simulink model "sympathetic_trip"  (R2019b)
settings: Solver=FixedStepAuto  StartTime=0.0  StopTime=1  FixedStep=0.0001  RelTol=1e-3
libraries: powerlib x16, powerlib_meascontrol x10, simulink x3, artemis x3
settings Model: Creator=nikgal-local  LastModifiedBy=nikgal-local
settings DataIOCC: ReturnWorkspaceOutputs=off
settings DebuggingCC: UnconnectedInputMsg=none  UnconnectedOutputMsg=none  UnconnectedLineMsg=none
settings RTWCC: GenCodeOnly=on

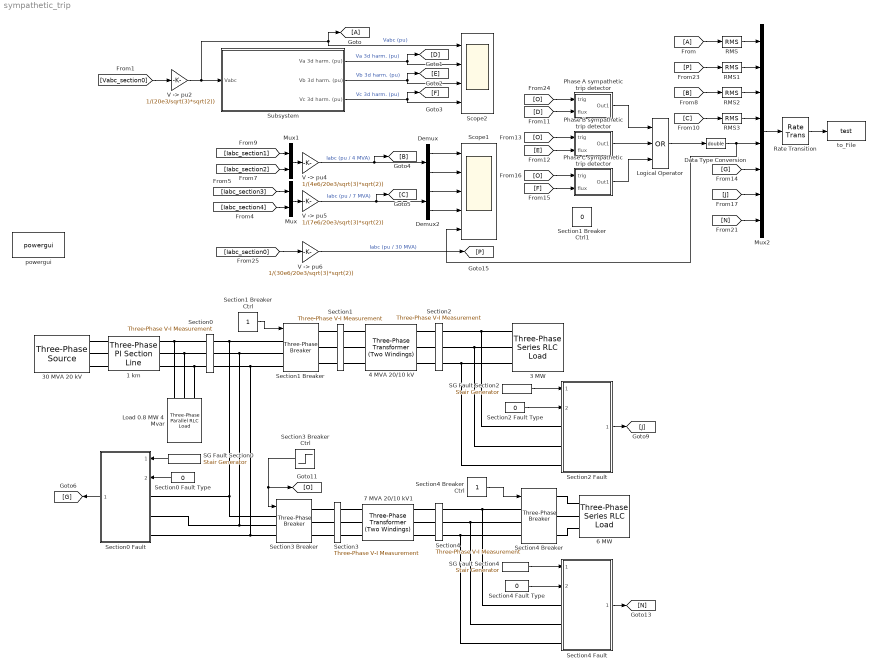
== system sympathetic_trip ==
  1 km : powerlib/Elements/Three-Phase PI Section Line  LConnTagsString=a|b|c  RConnTagsString=A|B|C  Frequency=50  Resistances=[ 0.01273 0.3864]  Inductances="[ 0.9337e-3  4.1264e-3]"  Capacitances=[12.74e-9 7.751e-9]  Length=1
      settings: SourceProductName=Simscape Electrical
  3 MW : powerlib/Elements/Three-Phase Series RLC Load  LConnTagsString=A|B|C  Configuration=Y (grounded)  NominalVoltage=10e3  Vabc=[1e3 1e3 1e3]  Vabcp=[1e3 1e3 1e3]  NominalFrequency=50  UnbalancedPower=off  ActivePower=3e6  InductivePower=0  CapacitivePower=0  Pabc=[10e3 9e3 11e3]  QLabc=[100 90 110]  QCabc=[100 90 110]  Pabcp=[10e3 9e3 11e3]  QLabcp=[100 90 110]  QCabcp=[100 90 110]  Measurements=None  LoadType=constant Z
      settings: SourceProductName=Simscape Electrical
  30 MVA 20 kV : powerlib/Electrical Sources/Three-Phase Source  InternalConnection=Yg  VoltagePhases=off  Voltage=20e3  PhaseAngle=15  Voltage_phases=[25e3 25e3 25e3]/sqrt(3)  PhaseAngles_phases=[0 -120 +120]  Frequency=50  NonIdealSource=on  SpecifyImpedance=off  Resistance=1.33  Inductance=35.3e-3  ShortCircuitLevel=30e6  BaseVoltage=20e3  XRratio=10  BusType=swing  Pref=10e3  Qref=0  Prefabc=[10e3, 10e3, 10e3]  Qrefabc=[0, 0, 0]  Qmin=-inf  Qmax=inf
      settings: SourceProductName=Simscape Electrical
  4 MVA 20/10 kV : powerlib/Elements/Three-Phase Transformer (Two Windings)  Winding1Connection=Yg  Winding2Connection=Yg  CoreType=Three single-phase transformers  SetSaturation=on  Hysteresis=off  DataFile='hysteresis'  SetInitialFlux=off  Measurements=None  UNITS=pu  NominalPower=[ 4e6 , 50 ]  Winding1=[ 20e3 , 0.05 , 0.08 ]  Winding2=[ 10e3 , 0.05 , 0.08 ]  Rm=500  Lm=500  L0=0.5  Saturation=[ 0,0 ; 0.0012,1.2 ; 1.0,1.45 ]  InitialFluxes=[-1.04733441543709 0.447873926928996 0.599252337980466]  BreakLoop=off  DiscreteSolver=Trapezoidal iterative  DataType=off  TransfoNumber=1
      settings: SourceProductName=Simscape Electrical
  6 MW : powerlib/Elements/Three-Phase Series RLC Load  LConnTagsString=A|B|C  Configuration=Y (grounded)  NominalVoltage=10e3  Vabc=[1e3 1e3 1e3]  Vabcp=[1e3 1e3 1e3]  NominalFrequency=50  UnbalancedPower=off  ActivePower=6e6  InductivePower=0  CapacitivePower=0  Pabc=[10e3 9e3 11e3]  QLabc=[100 90 110]  QCabc=[100 90 110]  Pabcp=[10e3 9e3 11e3]  QLabcp=[100 90 110]  QCabcp=[100 90 110]  Measurements=None  LoadType=constant Z
      settings: SourceProductName=Simscape Electrical
  7 MVA 20/10 kV1 : powerlib/Elements/Three-Phase Transformer (Two Windings)  Winding1Connection=Yg  Winding2Connection=Yg  CoreType=Three single-phase transformers  SetSaturation=on  Hysteresis=off  DataFile='hysteresis'  SetInitialFlux=on  Measurements=None  UNITS=pu  NominalPower=[ 7e6 , 50 ]  Winding1=[ 20e3 , 0.05 , 0.08 ]  Winding2=[ 10e3 , 0.05 , 0.08 ]  Rm=500  Lm=500  L0=0.5  Saturation=[ 0,0 ; 0.0012,1.2 ; 1.0,1.45 ]  InitialFluxes=[0.8 -0.4 0.4]  BreakLoop=off  DiscreteSolver=Trapezoidal iterative  DataType=off  TransfoNumber=1
      settings: SourceProductName=Simscape Electrical
  Data Type Conversion : DataTypeConversion  OutMin=[0]  OutMax=[1]  OutDataTypeStr=double
  Demux : Demux  Outputs=2
  Demux2 : Demux  Outputs=2
  Load 0.8 MW 4 Mvar : powerlib/Elements/Three-Phase Parallel RLC Load  LConnTagsString=A|B|C  Configuration=Y (grounded)  NominalVoltage=20e3  Vabc=[1e3 1e3 1e3]  Vabcp=[1e3 1e3 1e3]  NominalFrequency=50  UnbalancedPower=off  ActivePower=0.8e6  InductivePower=0  CapacitivePower=4e6  Pabc=[10e3 9e3 11e3]  QLabc=[100 90 110]  QCabc=[100 90 110]  Pabcp=[10e3 9e3 11e3]  QLabcp=[100 90 110]  QCabcp=[100 90 110]  Measurements=None  LoadType=constant Z
      settings: SourceProductName=Simscape Electrical
  Logical Operator : Logic  Operator=OR  Inputs=3  AllPortsSameDT=off  OutDataTypeStr=boolean
  Mux : Mux  Inputs=2
  Mux1 : Mux  Inputs=2
  Mux2 : Mux  Inputs=8
  Phase A sympathetic trip detector : Subsystem
  Phase B sympathetic trip detector : Subsystem
  Phase C sympathetic trip detector : Subsystem
  RMS{,1..3} (4 alike) : powerlib_meascontrol/Measurements/RMS  TrueRMS=on  Freq=50  RMSInit=1  Ts=0
      settings: SourceProductName=Simscape Electrical
  Rate Transition : RateTransition  OutPortSampleTime=0.0005
  SG Fault Section0 : powerlib_meascontrol/Pulse & Signal Generators/Stair Generator  t=[0, 0.5, 0.7]  e=[0, 1, 0]  Ts=0
      settings: SourceProductName=Simscape Electrical
  SG Fault Section2 : powerlib_meascontrol/Pulse & Signal Generators/Stair Generator  t=[0, 0.5, 0.7]  e=[0, 1, 0]  Ts=0
      settings: SourceProductName=Simscape Electrical
  SG Fault Section4 : powerlib_meascontrol/Pulse & Signal Generators/Stair Generator  t=[0, 0.5, 0.7]  e=[0, 1, 0]  Ts=0
      settings: SourceProductName=Simscape Electrical
  Scope1 : Scope  NumInputPorts=5
  Scope2 : Scope  NumInputPorts=4
  Section0 : powerlib/Measurements/Three-Phase V-I Measurement  VoltageMeasurement=phase-to-ground  SetLabelV=on  LabelV=Vabc_section0  Vpu=off  VpuLL=off  CurrentMeasurement=yes  SetLabelI=on  LabelI=Iabc_section0  Ipu=off  Pbase=100e6  Vbase=500e3  OutputType=Complex  PhasorSimulation=off  PSBequivalent=0
      settings: SourceProductName=Simscape Electrical
  Section0 Fault : Subsystem
  Section0 Fault Type : Constant  Value=0
  Section1 : powerlib/Measurements/Three-Phase V-I Measurement  VoltageMeasurement=phase-to-ground  SetLabelV=on  LabelV=Vabc_section1  Vpu=off  VpuLL=off  CurrentMeasurement=yes  SetLabelI=on  LabelI=Iabc_section1  Ipu=off  Pbase=100e6  Vbase=500e3  OutputType=Complex  PhasorSimulation=off  PSBequivalent=0
      settings: SourceProductName=Simscape Electrical
  Section1 Breaker : powerlib/Elements/Three-Phase Breaker  InitialState=closed  SwitchA=on  SwitchB=on  SwitchC=on  SwitchTimes=[0]  External=on  BreakerResistance=0.01  SnubberResistance=1e6  SnubberCapacitance=150e-6  Measurements=None
      settings: SourceProductName=Simscape Electrical
  Section1 Breaker Ctrl : Constant
  Section1 Breaker Ctrl1 : Constant  Value=0
  Section2 : powerlib/Measurements/Three-Phase V-I Measurement  VoltageMeasurement=no  SetLabelV=off  LabelV=Vabc  Vpu=off  VpuLL=off  CurrentMeasurement=yes  SetLabelI=on  LabelI=Iabc_section2  Ipu=off  Pbase=100e6  Vbase=500e3  OutputType=Complex  PhasorSimulation=off  PSBequivalent=0
      settings: SourceProductName=Simscape Electrical
  Section2 Fault : Subsystem
  Section2 Fault Type : Constant  Value=0
  Section3 : powerlib/Measurements/Three-Phase V-I Measurement  VoltageMeasurement=no  SetLabelV=off  LabelV=Vabc  Vpu=off  VpuLL=off  CurrentMeasurement=yes  SetLabelI=on  LabelI=Iabc_section3  Ipu=off  Pbase=100e6  Vbase=500e3  OutputType=Complex  PhasorSimulation=off  PSBequivalent=0
      settings: SourceProductName=Simscape Electrical
  Section3 Breaker : powerlib/Elements/Three-Phase Breaker  InitialState=open  SwitchA=on  SwitchB=on  SwitchC=on  SwitchTimes=[12/50]  External=on  BreakerResistance=0.01  SnubberResistance=1e6  SnubberCapacitance=150e-6  Measurements=None
      settings: SourceProductName=Simscape Electrical
  Section3 Breaker Ctrl : Step  Time=0.5  SampleTime=0
  Section4 : powerlib/Measurements/Three-Phase V-I Measurement  VoltageMeasurement=no  SetLabelV=off  LabelV=Vabc  Vpu=off  VpuLL=off  CurrentMeasurement=yes  SetLabelI=on  LabelI=Iabc_section4  Ipu=off  Pbase=100e6  Vbase=500e3  OutputType=Complex  PhasorSimulation=off  PSBequivalent=0
      settings: SourceProductName=Simscape Electrical
  Section4 Breaker : powerlib/Elements/Three-Phase Breaker  InitialState=closed  SwitchA=on  SwitchB=on  SwitchC=on  SwitchTimes=[12/50]  External=on  BreakerResistance=0.01  SnubberResistance=1e6  SnubberCapacitance=150e-6  Measurements=None
      settings: SourceProductName=Simscape Electrical
  Section4 Breaker Ctrl : Constant
  Section4 Fault : Subsystem
  Section4 Fault Type : Constant  Value=0
  Subsystem : Subsystem
  "V -> pu2" : Gain  Gain=1/(20e3/sqrt(3)*sqrt(2))  SaturateOnIntegerOverflow=on  OutDataTypeStr=Inherit: Same as input  ParamDataTypeStr=Inherit: Same as input
  "V -> pu4" : Gain  Gain=1/(4e6/20e3/sqrt(3)*sqrt(2))  SaturateOnIntegerOverflow=on  OutDataTypeStr=Inherit: Same as input  ParamDataTypeStr=Inherit: Same as input
  "V -> pu5" : Gain  Gain=1/(7e6/20e3/sqrt(3)*sqrt(2))  SaturateOnIntegerOverflow=on  OutDataTypeStr=Inherit: Same as input  ParamDataTypeStr=Inherit: Same as input
  "V -> pu6" : Gain  Gain=1/(30e6/20e3/sqrt(3)*sqrt(2))  SaturateOnIntegerOverflow=on  OutDataTypeStr=Inherit: Same as input  ParamDataTypeStr=Inherit: Same as input
  powergui : powerlib/powergui  Priority=1  SimulationMode=Discrete  SampleTime=0.0001  frequency=60  Iterations=50  frequencyindice=0  Pbase=100e6  ErrMax=1e-4  UnitsV=kV  UnitsW=MW  buscounter=0  FunctionMessages=off  echomessages=off  EnableUseOfTLC=off  CurrentSourceSwitches=off  DisableSnubberDevices=off  DisableRonSwitches=off  DisableVfSwitches=off  DisplayEquations=off  AutomaticDiscreteSolvers=off  SolverType=Tustin/Backward Euler (TBE)  Interpol=off  ExternalGateDelay=off  methode=off  Ts=100  x0status=blocks  SPID=on  SwTol=0  HookPort=off  NonlinearTolerance=1e-4  nMaxIteration=100  ContinueOnMaxIteration=off  RestoreLinks=warning  ResistiveCurrentMeasurement=off  Frange=[0:2:500]  Ylog=off  Xlog=on  ShowGrid=off  save=off  variable=ZData  structure=my_test_scope1  ZoomFFT=off  StartTime=0.33  cycles=4  DisplayStyle=1  fundamental=50  FreqAxis=on  MaxFrequency=1000  frequencyindicesteady=1  RmsSteady=1  display=off
      settings: SourceProductName=Simscape Electrical
  to_File : ToFile  Filename=test
  wires:
  "V -> pu2"/1 -> [A], Scope2/1, Subsystem/1(Vabc)  "Vabc (pu)"
  [Vabc_section0] -> "V -> pu2"/1
  Subsystem/1(Va 3d harm. (pu)) -> [D], Scope2/2  "Va 3d harm. (pu)"
  Subsystem/2(Vb 3d harm. (pu)) -> [E], Scope2/3  "Vb 3d harm. (pu)"
  Subsystem/3(Vc 3d harm. (pu)) -> [F], Scope2/4  "Vc 3d harm. (pu)"
  [Iabc_section3] -> Mux/1
  [Iabc_section4] -> Mux/2
  Mux/1 -> "V -> pu5"/1
  Mux1/1 -> "V -> pu4"/1
  "V -> pu4"/1 -> [B], Demux/1  "Iabc (pu / 4 MVA)"
  [Iabc_section1] -> Mux1/1
  [Iabc_section2] -> Mux1/2
  "V -> pu5"/1 -> [C], Demux2/1  "Iabc (pu / 7 MVA)"
  Demux/1 -> Scope1/1
  Demux/2 -> Scope1/2
  Demux2/1 -> Scope1/3
  Demux2/2 -> Scope1/4
  [A] -> RMS/1
  Section3 Breaker Ctrl/1 -> [O], Section3 Breaker/1
  Section4 Breaker Ctrl/1 -> Section4 Breaker/1
  "V -> pu6"/1 -> [P]  "Iabc (pu / 30 MVA)"
  [Iabc_section0] -> "V -> pu6"/1
  [P] -> RMS1/1
  [B] -> RMS2/1
  [C] -> RMS3/1
  [O] -> Phase A sympathetic trip detector/1(trig)
  [D] -> Phase A sympathetic trip detector/2(flux)
  [O] -> Phase B sympathetic trip detector/1(trig)
  [E] -> Phase B sympathetic trip detector/2(flux)
  [F] -> Phase C sympathetic trip detector/2(flux)
  [O] -> Phase C sympathetic trip detector/1(trig)
  Mux2/1 -> Rate Transition/1
  Rate Transition/1 -> to_File/1
  RMS/1 -> Mux2/1
  RMS1/1 -> Mux2/2
  RMS2/1 -> Mux2/3
  RMS3/1 -> Mux2/4
  Section1 Breaker Ctrl/1 -> Section1 Breaker/1
  Phase A sympathetic trip detector/1(Out1) -> Logical Operator/1
  Phase B sympathetic trip detector/1(Out1) -> Logical Operator/2
  Phase C sympathetic trip detector/1(Out1) -> Logical Operator/3
  [G] -> Mux2/6
  [J] -> Mux2/7
  [N] -> Mux2/8
  Logical Operator/1 -> Data Type Conversion/1
  Data Type Conversion/1 -> Scope1/5, Mux2/5
  SG Fault Section2/1 -> Section2 Fault/1(activate fault)
  Section2 Fault/1(fault status) -> [J]
  Section2 Fault Type/1 -> Section2 Fault/2(fault type)
  SG Fault Section0/1 -> Section0 Fault/1(activate fault)
  Section0 Fault Type/1 -> Section0 Fault/2(fault type)
  Section0 Fault/1(fault status) -> [G]
  Section4 Fault/1(fault status) -> [N]
  Section4 Fault Type/1 -> Section4 Fault/2(fault type)
  SG Fault Section4/1 -> Section4 Fault/1(activate fault)
  connections:
  30 MVA 20 kV/RConn2 -- 1 km/LConn2
  30 MVA 20 kV/RConn1 -- 1 km/LConn1
  30 MVA 20 kV/RConn3 -- 1 km/LConn3
  Section1 Breaker/LConn1 -- Section3 Breaker/LConn1 -- Section0 Fault/LConn1 -- Section0/RConn1
  Section3 Breaker/LConn2 -- Section0 Fault/LConn2 -- Section1 Breaker/LConn2 -- Section0/RConn2
  Section1 Breaker/LConn3 -- Section0 Fault/LConn3 -- Section3 Breaker/LConn3 -- Section0/RConn3
  4 MVA 20/10 kV/RConn1 -- Section2/LConn1
  4 MVA 20/10 kV/RConn2 -- Section2/LConn2
  4 MVA 20/10 kV/RConn3 -- Section2/LConn3
  3 MW/LConn1 -- Section2 Fault/LConn1 -- Section2/RConn1
  3 MW/LConn2 -- Section2 Fault/LConn2 -- Section2/RConn2
  3 MW/LConn3 -- Section2 Fault/LConn3 -- Section2/RConn3
  Section3 Breaker/RConn1 -- Section3/LConn1
  Section3 Breaker/RConn2 -- Section3/LConn2
  Section3 Breaker/RConn3 -- Section3/LConn3
  7 MVA 20/10 kV1/LConn1 -- Section3/RConn1
  7 MVA 20/10 kV1/LConn2 -- Section3/RConn2
  7 MVA 20/10 kV1/LConn3 -- Section3/RConn3
  7 MVA 20/10 kV1/RConn1 -- Section4/LConn1
  7 MVA 20/10 kV1/RConn2 -- Section4/LConn2
  7 MVA 20/10 kV1/RConn3 -- Section4/LConn3
  Section4 Breaker/LConn3 -- Section4 Fault/LConn3 -- Section4/RConn3
  6 MW/LConn3 -- Section4 Breaker/RConn3
  6 MW/LConn2 -- Section4 Breaker/RConn2
  6 MW/LConn1 -- Section4 Breaker/RConn1
  Section4 Breaker/LConn2 -- Section4 Fault/LConn2 -- Section4/RConn2
  Section4 Breaker/LConn1 -- Section4 Fault/LConn1 -- Section4/RConn1
  Section1/RConn1 -- 4 MVA 20/10 kV/LConn1
  Section1/RConn2 -- 4 MVA 20/10 kV/LConn2
  Section1/RConn3 -- 4 MVA 20/10 kV/LConn3
  Section1 Breaker/RConn1 -- Section1/LConn1
  Section1 Breaker/RConn2 -- Section1/LConn2
  Section1 Breaker/RConn3 -- Section1/LConn3
  Section0/LConn3 -- Load 0.8 MW 4 Mvar/LConn3 -- 1 km/RConn3
  Section0/LConn2 -- Load 0.8 MW 4 Mvar/LConn2 -- 1 km/RConn2
  Section0/LConn1 -- Load 0.8 MW 4 Mvar/LConn1 -- 1 km/RConn1

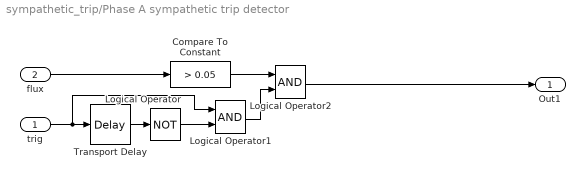
== system sympathetic_trip/Phase A sympathetic trip detector ==
  trig : Inport
  flux : Inport  Port=2
  Compare To Constant : simulink/Logic and Bit Operations/Compare To Constant  relop=>  const=0.05  OutDataTypeStr=boolean
  Logical Operator : Logic  Operator=NOT  AllPortsSameDT=off  OutDataTypeStr=boolean
  Logical Operator1 : Logic  AllPortsSameDT=off  OutDataTypeStr=boolean
  Logical Operator2 : Logic  AllPortsSameDT=off  OutDataTypeStr=boolean
  Transport Delay : TransportDelay  DelayTime=0.4  BufferSize=4096
  Out1 : Outport
  wires:
  Transport Delay/1 -> Logical Operator/1
  Logical Operator/1 -> Logical Operator1/2
  trig/1 -> Logical Operator1/1, Transport Delay/1
  flux/1 -> Compare To Constant/1
  Compare To Constant/1 -> Logical Operator2/1
  Logical Operator2/1 -> Out1/1
  Logical Operator1/1 -> Logical Operator2/2

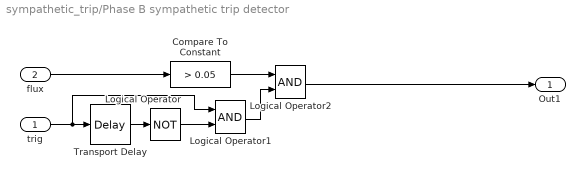
== system sympathetic_trip/Phase B sympathetic trip detector ==
  trig : Inport
  flux : Inport  Port=2
  Compare To Constant : simulink/Logic and Bit Operations/Compare To Constant  relop=>  const=0.05  OutDataTypeStr=boolean
  Logical Operator : Logic  Operator=NOT  AllPortsSameDT=off  OutDataTypeStr=boolean
  Logical Operator1 : Logic  AllPortsSameDT=off  OutDataTypeStr=boolean
  Logical Operator2 : Logic  AllPortsSameDT=off  OutDataTypeStr=boolean
  Transport Delay : TransportDelay  DelayTime=0.4  BufferSize=4096
  Out1 : Outport
  wires:
  Transport Delay/1 -> Logical Operator/1
  Logical Operator/1 -> Logical Operator1/2
  trig/1 -> Logical Operator1/1, Transport Delay/1
  flux/1 -> Compare To Constant/1
  Compare To Constant/1 -> Logical Operator2/1
  Logical Operator2/1 -> Out1/1
  Logical Operator1/1 -> Logical Operator2/2

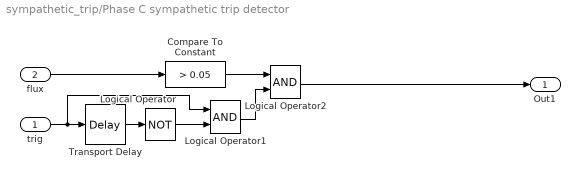
== system sympathetic_trip/Phase C sympathetic trip detector ==
  trig : Inport
  flux : Inport  Port=2
  Compare To Constant : simulink/Logic and Bit Operations/Compare To Constant  relop=>  const=0.05  OutDataTypeStr=boolean
  Logical Operator : Logic  Operator=NOT  AllPortsSameDT=off  OutDataTypeStr=boolean
  Logical Operator1 : Logic  AllPortsSameDT=off  OutDataTypeStr=boolean
  Logical Operator2 : Logic  AllPortsSameDT=off  OutDataTypeStr=boolean
  Transport Delay : TransportDelay  DelayTime=0.4  BufferSize=4096
  Out1 : Outport
  wires:
  Transport Delay/1 -> Logical Operator/1
  Logical Operator/1 -> Logical Operator1/2
  trig/1 -> Logical Operator1/1, Transport Delay/1
  flux/1 -> Compare To Constant/1
  Compare To Constant/1 -> Logical Operator2/1
  Logical Operator2/1 -> Out1/1
  Logical Operator1/1 -> Logical Operator2/2

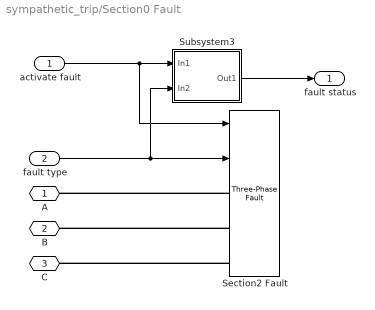
== system sympathetic_trip/Section0 Fault ==
  activate fault : Inport
  fault type : Inport  Port=2
  Section2 Fault : artemis/Tools /Custom Models/Three-Phase Fault  FaultA=on  FaultB=on  FaultC=on  FaultResistance=1  GroundFault=on  GroundResistance=0.001  External=on  SwitchStatus=[1 0 1 0 ]  SwitchTimes=[ 5/50 7/50 15/50 19/50]  InitialStates=[0 0 1]  SnubberResistance=1e6  SnubberCapacitance=inf  Measurements=None
  Subsystem3 : Subsystem
  A : PMIOPort  Side=Left
  B : PMIOPort  Port=2  Side=Left
  C : PMIOPort  Port=3  Side=Left
  fault status : Outport
  wires:
  activate fault/1 -> Subsystem3/1(In1), Section2 Fault/1
  fault type/1 -> Subsystem3/2(In2), Section2 Fault/2
  Subsystem3/1(Out1) -> fault status/1
  connections:
  Section2 Fault/LConn3 -- C/RConn1
  Section2 Fault/LConn1 -- A/RConn1
  Section2 Fault/LConn2 -- B/RConn1

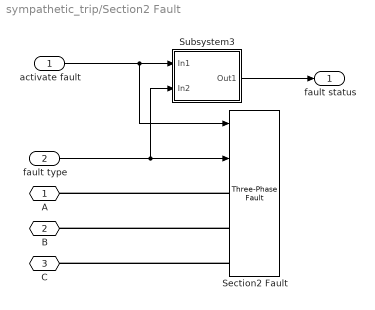
== system sympathetic_trip/Section2 Fault ==
  activate fault : Inport
  fault type : Inport  Port=2
  Section2 Fault : artemis/Tools /Custom Models/Three-Phase Fault  FaultA=on  FaultB=on  FaultC=on  FaultResistance=1  GroundFault=on  GroundResistance=0.001  External=on  SwitchStatus=[1 0 1 0 ]  SwitchTimes=[ 5/50 7/50 15/50 19/50]  InitialStates=[0 0 1]  SnubberResistance=1e6  SnubberCapacitance=inf  Measurements=None
  Subsystem3 : Subsystem
  A : PMIOPort  Side=Left
  B : PMIOPort  Port=2  Side=Left
  C : PMIOPort  Port=3  Side=Left
  fault status : Outport
  wires:
  activate fault/1 -> Subsystem3/1(In1), Section2 Fault/1
  fault type/1 -> Subsystem3/2(In2), Section2 Fault/2
  Subsystem3/1(Out1) -> fault status/1
  connections:
  Section2 Fault/LConn3 -- C/RConn1
  Section2 Fault/LConn1 -- A/RConn1
  Section2 Fault/LConn2 -- B/RConn1

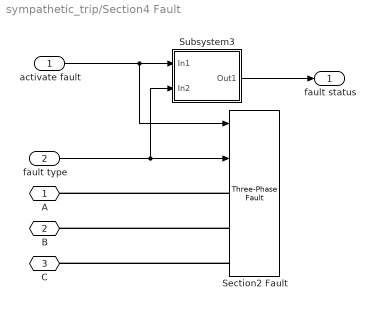
== system sympathetic_trip/Section4 Fault ==
  activate fault : Inport
  fault type : Inport  Port=2
  Section2 Fault : artemis/Tools /Custom Models/Three-Phase Fault  FaultA=on  FaultB=on  FaultC=on  FaultResistance=1  GroundFault=on  GroundResistance=0.001  External=on  SwitchStatus=[1 0 1 0 ]  SwitchTimes=[ 5/50 7/50 15/50 19/50]  InitialStates=[0 0 1]  SnubberResistance=1e6  SnubberCapacitance=inf  Measurements=None
  Subsystem3 : Subsystem
  A : PMIOPort  Side=Left
  B : PMIOPort  Port=2  Side=Left
  C : PMIOPort  Port=3  Side=Left
  fault status : Outport
  wires:
  activate fault/1 -> Subsystem3/1(In1), Section2 Fault/1
  fault type/1 -> Subsystem3/2(In2), Section2 Fault/2
  Subsystem3/1(Out1) -> fault status/1
  connections:
  Section2 Fault/LConn3 -- C/RConn1
  Section2 Fault/LConn1 -- A/RConn1
  Section2 Fault/LConn2 -- B/RConn1

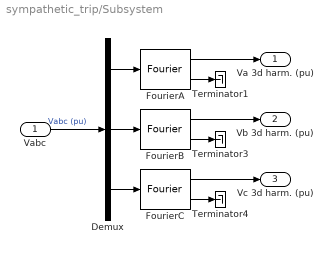
== system sympathetic_trip/Subsystem ==
  Vabc : Inport
  Demux : Demux  Outputs=3
  FourierA : powerlib_meascontrol/Measurements/Fourier  Freq=50  n=3  InInit=[0, 0]  Ts=0
      settings: SourceProductName=Simscape Electrical
  FourierB : powerlib_meascontrol/Measurements/Fourier  Freq=50  n=3  InInit=[0, 0]  Ts=0
      settings: SourceProductName=Simscape Electrical
  FourierC : powerlib_meascontrol/Measurements/Fourier  Freq=50  n=3  InInit=[0, 0]  Ts=0
      settings: SourceProductName=Simscape Electrical
  Terminator1 : Terminator
  Terminator3 : Terminator
  Terminator4 : Terminator
  Va 3d harm. (pu) : Outport
  Vb 3d harm. (pu) : Outport  Port=2
  Vc 3d harm. (pu) : Outport  Port=3
  wires:
  FourierA/1 -> Va 3d harm. (pu)/1
  FourierB/2 -> Terminator3/1
  FourierA/2 -> Terminator1/1
  FourierC/2 -> Terminator4/1
  FourierC/1 -> Vc 3d harm. (pu)/1
  FourierB/1 -> Vb 3d harm. (pu)/1
  Demux/2 -> FourierB/1
  Demux/1 -> FourierA/1
  Demux/3 -> FourierC/1
  Vabc/1 -> Demux/1  "Vabc (pu)"

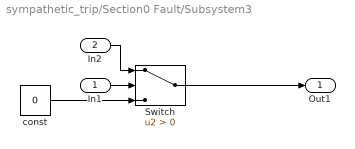
== system sympathetic_trip/Section0 Fault/Subsystem3 ==
  In1 : Inport
  In2 : Inport  Port=2
  Switch : Switch  Criteria=u2 > Threshold
  const : Constant  Value=0
  Out1 : Outport
  wires:
  const/1 -> Switch/3
  Switch/1 -> Out1/1
  In2/1 -> Switch/1
  In1/1 -> Switch/2

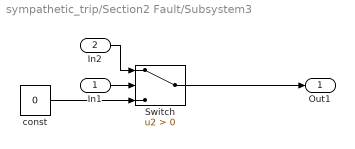
== system sympathetic_trip/Section2 Fault/Subsystem3 ==
  In1 : Inport
  In2 : Inport  Port=2
  Switch : Switch  Criteria=u2 > Threshold
  const : Constant  Value=0
  Out1 : Outport
  wires:
  const/1 -> Switch/3
  Switch/1 -> Out1/1
  In2/1 -> Switch/1
  In1/1 -> Switch/2

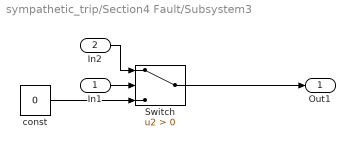
== system sympathetic_trip/Section4 Fault/Subsystem3 ==
  In1 : Inport
  In2 : Inport  Port=2
  Switch : Switch  Criteria=u2 > Threshold
  const : Constant  Value=0
  Out1 : Outport
  wires:
  const/1 -> Switch/3
  Switch/1 -> Out1/1
  In2/1 -> Switch/1
  In1/1 -> Switch/2
